simulink model "Test_model"  (R2024a)
settings: Solver=VariableStepAuto  StartTime=0.0  StopTime=inf  RelTol=1e-3
undefined symbols (not defined in the file or in its folder): X, Y, Z
libraries: sm_lib x63, nesl_utility x19
(part 1 of 2)
settings Model: Creator=pimna  LastModifiedBy=pimna

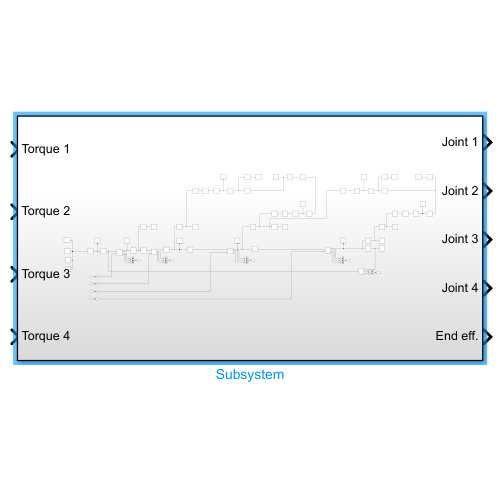
[thumbnail: Simulink's stored preview of the top-level diagram]
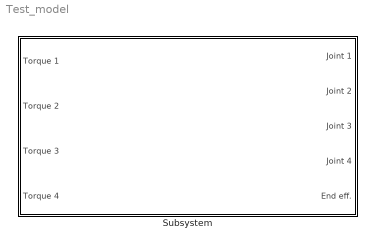
== system Test_model ==
  Subsystem : Subsystem
